simulink model "chap4_3"  (Simulink 5.1)
settings: Solver=ode45  StartTime=0.0  StopTime=3  RelTol=1e-3
libraries: fuzblock x1
settings Model: LastModifiedBy=Administrator  BooleanDataType=on  ProdHWDeviceType=Microprocessor

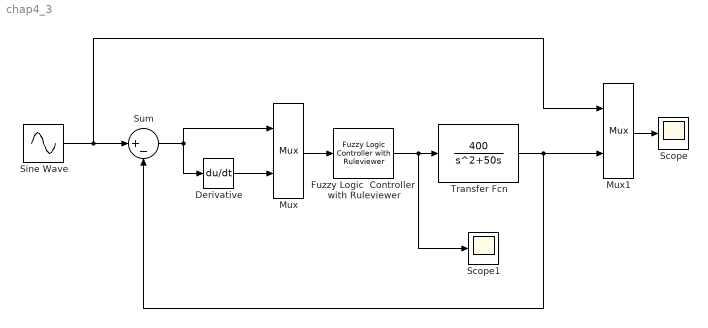
== system chap4_3 ==
  Derivative : Derivative
  Fuzzy Logic  Controller  with Ruleviewer : fuzblock/Fuzzy Logic  Controller  with Ruleviewer  fismatrix=a2  Ts=2
      link override Fuzzy Logic Controller: fis=a2
  Mux : Mux  Inputs=2
  Mux1 : Mux  Inputs=2
  Scope : Scope
      settings: TimeRange=3  YMin=0.1  YMax=0.5  MaxDataPoints=50000
  Scope1 : Scope
      settings: YMin=-20  YMax=40
  Sine Wave : Sin  Amplitude=0.5  Frequency=10  SampleTime=0
  Sum : Sum  Inputs=|+-  SaturateOnIntegerOverflow=on  InputSameDT=on
  Transfer Fcn : TransferFcn  Numerator=[400]  Denominator=[1 50 0]
  wires:
  Mux/1 -> Fuzzy Logic  Controller  with Ruleviewer/1
  Derivative/1 -> Mux/2
  Sum/1 -> Mux/1, Derivative/1
  Sine Wave/1 -> Sum/1, Mux1/1
  Mux1/1 -> Scope/1
  Transfer Fcn/1 -> Mux1/2, Sum/2
  Fuzzy Logic  Controller  with Ruleviewer/1 -> Transfer Fcn/1, Scope1/1
